simulink model "dc_motor_sim_simulink"  (R2019a)
settings: Solver=ode45  StartTime=0.0  StopTime=50.0  RelTol=1e-3  EnableMultiTasking=on
values from neighbouring files (symbols this model uses):
  J = 0.010    (= 0.01)    [dc_motor_simulink_modelling.m]
  K_e = 0.24+0.0080    (= 0.248)    [dc_motor_simulink_modelling.m]
  K_t = 0.36    [dc_motor_simulink_modelling.m]
  L_a = 0.00010    (= 0.0001)    [dc_motor_simulink_modelling.m]
  m3 = 0.00215055254478    [data_workspace.mat]    (also in p.m = constant3(1))
  m4 = 0.000906699781425    [data_workspace.mat]    (also in p.m = constant4(1))
  m_p1 = 0.00317019595645    [data_workspace.mat]    (also in p.m = constant_p1(1))
  m_p2 = 0.00218886821705    [data_workspace.mat]    (also in p.m = constant_p2(1))
  m_p3 = 0.00103611475607    [data_workspace.mat]    (also in p.m = constant_p3(1))
  R_a = 3.4997    [dc_motor_simulink_modelling.m]
  rd = (pi/30)    (= 0.10471975512)    [dc_motor_simulink_modelling.m]
settings Model: Creator=NewUser  LastModifiedBy=fotoyis
settings DataIOCC: LimitDataPoints=on  SaveFormat=Array  ReturnWorkspaceOutputs=off
settings OptimizationCC: LifeSpan=inf
settings DebuggingCC: SFUnexpectedBacktrackingDiag=warning  SFNoUnconditionalDefaultTransitionDiag=warning  SFExecutionAtInitializationDiag=none  ArithmeticOperatorsInVariantConditions=warning
settings HardwareCC: ProdBitPerPointer=32  ProdBitPerSizeT=32  ProdBitPerPtrDiffT=32  ProdLargestAtomicFloat=None  ProdIntDivRoundTo=Undefined  ProdEndianess=Unspecified  ProdWordSize=32  ProdHWDeviceType=32-bit Generic
settings ModelReferenceCC: PropagateSignalLabelsOutOfModel=off
settings SFSimCC: SimUseLocalCustomCode=off
settings RTWCC: RTWUseLocalCustomCode=off
settings CodeAppCC: StateflowObjectComments=on
settings GRTTargetCC: TargetLangStandard=C89/C90 (ANSI)  GeneratePreprocessorConditionals=Disable all
settings ConfigComp: CovMetricSettings=dw  CovHtmlReporting=on  CovSaveCumulativeToWorkspaceVar=on  CovSaveSingleToWorkspaceVar=on  CovExternalEMLEnable=off

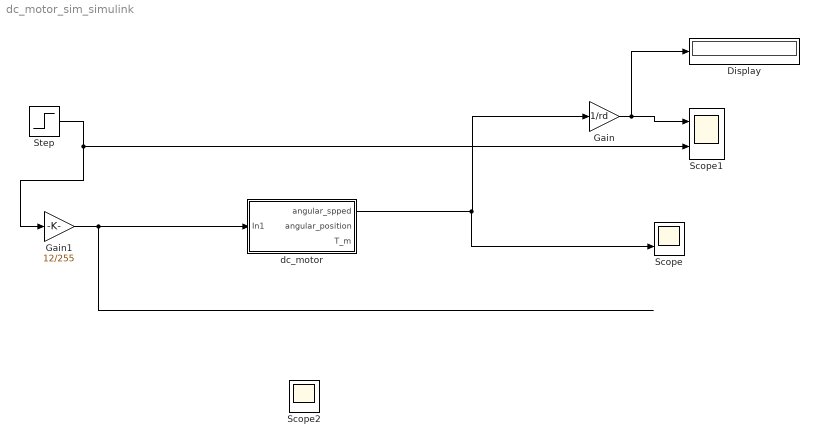
== system dc_motor_sim_simulink ==
  Display : Display
  Gain : Gain  Gain=1/rd
  Gain1 : Gain  Gain=12/255
  Scope : Scope  NumInputPorts=2
  Scope1 : Scope  NumInputPorts=2
  Scope2 : Scope
  Step : Step  Time=0  After=50  SampleTime=0
  dc_motor : Subsystem
  wires:
  Gain1/1 -> dc_motor/1(In1)
  Gain/1 -> Display/1, Scope1/1
  dc_motor/1(angular_spped) -> Scope/2, Gain/1
  Step/1 -> Gain1/1, Scope1/2

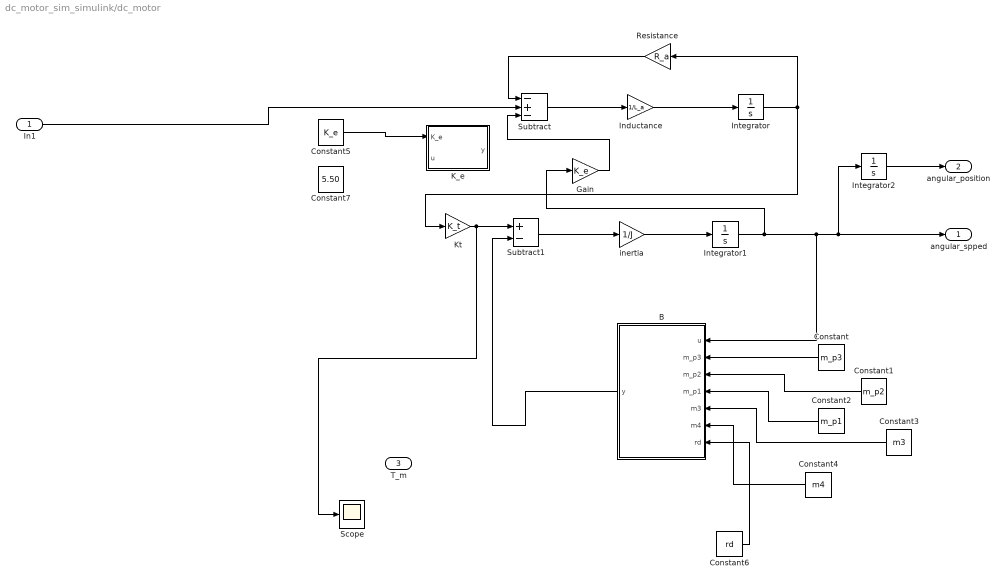
== system dc_motor_sim_simulink/dc_motor ==
  In1 : Inport
  B : MATLAB Function  TreatAsAtomicUnit=on
  Constant : Constant  Value=m_p3
  Constant1 : Constant  Value=m_p2
  Constant2 : Constant  Value=m_p1
  Constant3 : Constant  Value=m3
  Constant4 : Constant  Value=m4
  Constant5 : Constant  Value=K_e
  Constant6 : Constant  Value=rd
  Constant7 : Constant  Value=5.50
  Gain : Gain  Gain=K_e
  Inductance : Gain  Gain=1/L_a
  Integrator : Integrator
  Integrator1 : Integrator
  Integrator2 : Integrator
  K_e : MATLAB Function  TreatAsAtomicUnit=on
  "Kt " : Gain  Gain=K_t
  Resistance : Gain  Gain=R_a
  Scope : Scope
  Subtract : Sum  Inputs=-+-
  Subtract1 : Sum  Inputs=+-
  inertia : Gain  Gain=1/J
  angular_spped : Outport
  angular_position : Outport  Port=2
  T_m : Outport  Port=3
  wires:
  Integrator/1 -> "Kt "/1, Resistance/1
  Constant4/1 -> B/6(m4)
  Inductance/1 -> Integrator/1
  Constant3/1 -> B/5(m3)
  B/1(y) -> Subtract1/2
  Constant2/1 -> B/4(m_p1)
  Constant1/1 -> B/3(m_p2)
  Subtract1/1 -> inertia/1
  Resistance/1 -> Subtract/1
  inertia/1 -> Integrator1/1
  Subtract/1 -> Inductance/1
  Integrator2/1 -> angular_position/1
  Constant/1 -> B/2(m_p3)
  "Kt "/1 -> Scope/1, Subtract1/1
  In1/1 -> Subtract/2
  Integrator1/1 -> Gain/1, B/1(u), Integrator2/1, angular_spped/1
  Constant6/1 -> B/7(rd)
  Constant5/1 -> K_e/1(K_e)
  Gain/1 -> Subtract/3

== matlab function dc_motor_sim_simulink/dc_motor/K_e ==
  data: K_e input; u input; y output
function y = fcn(K_e, u)


%         if((u<-43*rd)&&(u>-50))
%             y_ = 0.373;
%         elseif((u>=50*rd)&&(u<74*rd))
%             y_ = 0.448;
%         elseif((u>=74*rd)&&(u<=98*rd))
%             y_ = 0.549;
%         elseif((u>98*rd)&&(u<=131*rd))
%             y_ = 0.653;
%         elseif((u>-131*rd)&&(u<=-150*rd))
%             y_ = 0.728;
       if((u >5)&&(u <9))
           y_ = K_e*u;
%        elseif((u>96*rd)&&(u<117*rd))
%            y_ = 0.21;
%        elseif((u>117*rd)&&(u<151*rd))
%            y_ = 0.189;
%        elseif((u >152*rd)&&(u < 171*rd))
%           y_ = 0.18;
%        else
%            y_ = 0.24;
       else
           y_ = 0;
       end
        
y = y_;

== matlab function dc_motor_sim_simulink/dc_motor/B ==
  data: u input; y output; m_p3 input; m_p2 input; m_p1 input; m3 input; m4 input; rd input
function y = fcn(u,m_p3,m_p2,m_p1,m3, m4, rd)
   % y_ = 0;
   
     if((u>0.0001*rd) &&(u<40*rd))
            y_ = -0.0378*u+0.6;
     elseif((u > -43*rd)&&(u<-0.0001*rd))
        y_ = -0.037*u-0.6;
     elseif((u >-150*rd)&&(u<-95*rd))
         y_ = m_p3*u-0.4801;
     elseif((u>-91*rd)&&(u<-74*rd))
         y_ =  m_p2*u-0.362;
             
     elseif((u>-71*rd)&&(u<-43*rd))
          y_ = m_p1*u-0.2877;
             
     elseif((u > 40*rd)&&(u <= 91*rd))
          y_ =  m3*u + 0.3271;
              
     elseif((u >91*rd)&&(u < 180*rd))
                  
          y_ =  m4*u + 0.4486;
     else
         y_ = 0.6;
     end
     
y = y_;
